simulink model "mympc"  (R2022a)
settings: Solver=VariableStepAuto  StartTime=0.0  StopTime=10.0  RelTol=1e-3
settings Model: Creator=mati  LastModifiedBy=mati

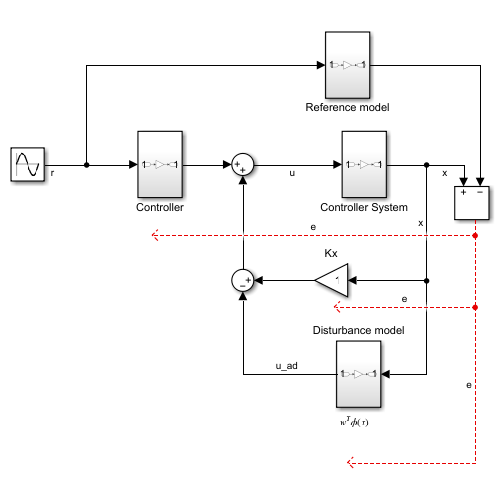
[thumbnail: Simulink's stored preview of the top-level diagram]
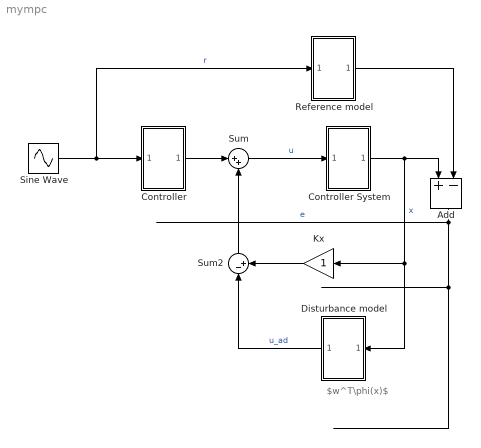
== system mympc ==
  note: $w^T\phi(x)$
  Add : Sum  Inputs=+-
  Controller : Subsystem
  Controller System : Subsystem
  Disturbance model : Subsystem
  Kx : Gain
  Reference model : Subsystem
  Sine Wave : Sin  SampleTime=0
  Sum : Sum  Inputs=|++
  Sum2 : Sum  Inputs=|-+
  wires:
  Sine Wave/1 -> Reference model/1(In1), Controller/1(In1)  "r"
  Controller/1(Out1) -> Sum/1
  Sum2/1 -> Sum/2
  Sum/1 -> Controller System/1(In1)  "u"
  Controller System/1(Out1) -> Disturbance model/1(In1), Kx/1, Add/1  "x"
  Reference model/1(Out1) -> Add/2
  Kx/1 -> Sum2/2
  Disturbance model/1(Out1) -> Sum2/1  "u_ad"
  Add/1 -> ?  "e"

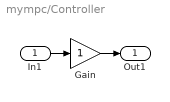
== system mympc/Controller ==
  In1 : Inport
  Gain : Gain
  Out1 : Outport
  wires:
  In1/1 -> Gain/1
  Gain/1 -> Out1/1

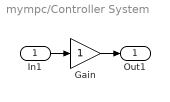
== system mympc/Controller System ==
  In1 : Inport
  Gain : Gain
  Out1 : Outport
  wires:
  In1/1 -> Gain/1
  Gain/1 -> Out1/1

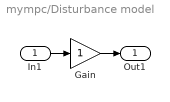
== system mympc/Disturbance model ==
  In1 : Inport
  Gain : Gain
  Out1 : Outport
  wires:
  In1/1 -> Gain/1
  Gain/1 -> Out1/1

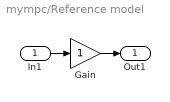
== system mympc/Reference model ==
  In1 : Inport
  Gain : Gain
  Out1 : Outport
  wires:
  In1/1 -> Gain/1
  Gain/1 -> Out1/1
